simulink model "whatchman"  (R2013b)
settings: Solver=ode45  StartTime=0.0  StopTime=10  RelTol=1e-3
libraries: simulink_extras x4
settings Model: Creator=Maksimus  LastModifiedBy=Maksimus

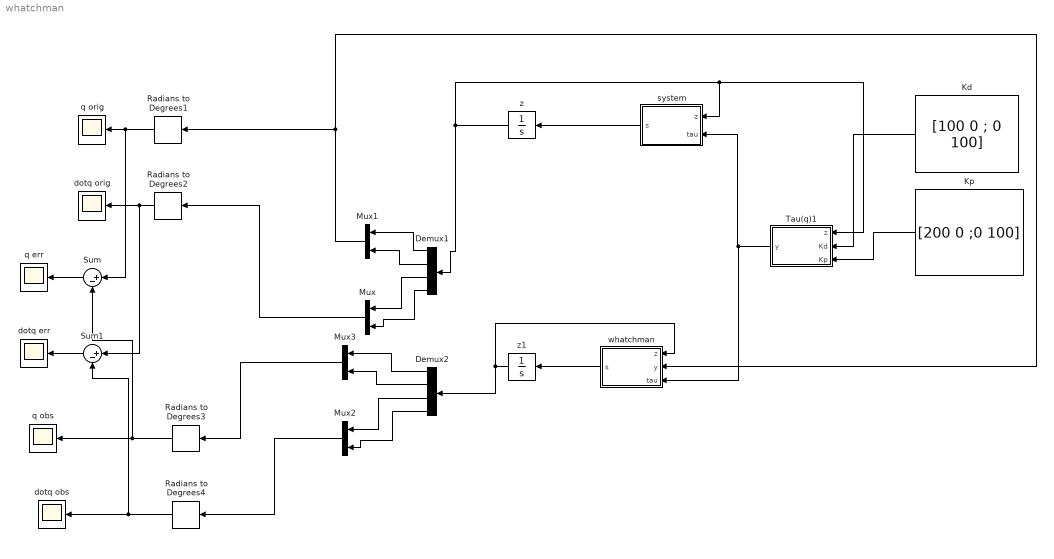
== system whatchman ==
  Demux1 : Demux
  Demux2 : Demux
  Kd : Constant  Value=[100 0 ; 0 100]
  "Kp " : Constant  Value=[200 0 ;0 100]
  Mux{,1..3} (4 alike) : Mux  Inputs=2
  Radians to Degrees{1..4} (4 alike) : simulink_extras/Transformations/Radians to Degrees
  Sum : Sum  Inputs=|+-
  Sum1 : Sum  Inputs=|+-
  Tau(q)1 : MATLAB Function  TreatAsAtomicUnit=on
  dotq err : Scope
      settings: YMin=0  YMax=30000  SaveName=ScopeData4
  dotq obs : Scope
      settings: YMin=0  YMax=30000
  dotq orig : Scope
      settings: YMin=0  YMax=30000  SaveName=ScopeData3
  q err : Scope
      settings: SaveName=ScopeData5
  q obs : Scope
  q orig : Scope
      settings: SaveName=ScopeData2
  system : MATLAB Function  TreatAsAtomicUnit=on
  whatchman : MATLAB Function  TreatAsAtomicUnit=on
  z : Integrator  InitialCondition=[0;0;0;0]  IgnoreLimit=on
  z1 : Integrator  InitialCondition=[-pi/2;0;0;0]  IgnoreLimit=on
  wires:
  Kd/1 -> Tau(q)1/2(Kd)
  z/1 -> Tau(q)1/1(z), system/1(z), Demux1/1
  Mux/1 -> Radians to Degrees2/1
  Demux1/1 -> Mux1/1
  Mux1/1 -> whatchman/2(y), Radians to Degrees1/1
  Radians to Degrees1/1 -> Sum/1, q orig/1
  Demux1/4 -> Mux/2
  Demux1/3 -> Mux/1
  system/1(s) -> z/1
  Tau(q)1/1(y) -> whatchman/3(tau), system/2(tau)
  "Kp "/1 -> Tau(q)1/3(Kp)
  Radians to Degrees2/1 -> Sum1/1, dotq orig/1
  Demux1/2 -> Mux1/2
  whatchman/1(s) -> z1/1
  z1/1 -> whatchman/1(z), Demux2/1
  Mux2/1 -> Radians to Degrees4/1
  Demux2/1 -> Mux3/1
  Mux3/1 -> Radians to Degrees3/1
  Radians to Degrees3/1 -> Sum/2, q obs/1
  Demux2/4 -> Mux2/2
  Demux2/3 -> Mux2/1
  Radians to Degrees4/1 -> Sum1/2, dotq obs/1
  Demux2/2 -> Mux3/2
  Sum1/1 -> dotq err/1
  Sum/1 -> q err/1

== matlab function whatchman/whatchman ==
  data: z input; y input; s output; tau input
function s = fcn(z,y,tau)
%задаем систему
m1 = 1; 
m2 = 1;
lc1 = 1;
lc2 = 2;
I1 = 0.12;
I2 = 0.12;
l1 = 1;
l2 = 1;
g=10;
m = [m1;m2];
lc = [lc1;lc2];
I = [I1;I2];
l = [l1;l2];
q = z(1:2);
dotq =z(3:4);

theta = [m(1)*lc(1)^2 + m(2)*l(1)^2 + I(1); m(2) * lc(2)^2 + I(2); m(2)*l(1)*lc(2); m(1)*lc(1) + m(2)*l(1); m(2)*lc(2)]; 

H = [theta(1) + theta(2) + 2 * theta(3)*cos(q(2)), theta(2) + theta(3) * cos(q(2));
    theta(2) + theta(3) * cos(q(2)), theta(2)]; 

C = [-theta(3) * sin(q(2)) * dotq(2), -theta(3) * sin(q(2)) * dotq(2) - theta(3) * sin(q(2)) * dotq(1);
    theta(3) * sin(q(2)) * dotq(1), 0];

G = [ theta(4) * g * cos(q(1)) + theta(5) * g * cos(q(1) + q(2)); theta(5) * g * cos(q(1) + q(2))]; %nonhorizontal robotarm
%конец задания системы


g1=15; %две константы, для того чтобы ошибка убывала
g2 = 210;

qcorrection =  g1* (y - q); %поправка для вектора углов
dotqcorrection =  g2*(y - q); %поправка для вектора скоростей
InvH = H^(-1);
InvHC = InvH * C;
InvHG = InvH * G;
tmpsys = - InvHC * dotq - InvHG + InvH*tau;
sys = [dotq + qcorrection ;tmpsys + dotqcorrection ]; 

s = sys;

== matlab function whatchman/system ==
  data: z input; s output; tau input
function s = fcn(z,tau)
%global linA linB linConst
%s = linA * z + linB * u + linConst;
m1 = 1;
m2 = 1;
lc1 = 1;
lc2 = 2;
I1 = 0.12;
I2 = 0.12;
l1 = 1;
l2 = 1;
g=10;

m = [m1;m2];
lc = [lc1;lc2];
I = [I1;I2];
l = [l1;l2];
dotq = z(3:4);
q = z(1:2);
theta = [m(1)*lc(1)^2 + m(2)*l(1)^2 + I(1); m(2) * lc(2)^2 + I(2); m(2)*l(1)*lc(2); m(1)*lc(1) + m(2)*l(1); m(2)*lc(2)]; 

H = [theta(1) + theta(2) + 2 * theta(3)*cos(q(2)), theta(2) + theta(3) * cos(q(2));
    theta(2) + theta(3) * cos(q(2)), theta(2)]; %is symmetrie, positive definite for all q

%H(q) - 2C(q, dotq) is a skew-syrnmetric matrix

C = [-theta(3) * sin(q(2)) * dotq(2), -theta(3) * sin(q(2)) * dotq(2) - theta(3) * sin(q(2)) * dotq(1);
    theta(3) * sin(q(2)) * dotq(1), 0];

G = [ theta(4) * g * cos(q(1)) + theta(5) * g * cos(q(1) + q(2)); theta(5) * g * cos(q(1) + q(2))]; %nonhorizontal robotarm


InvH = H^(-1);
InvHC = InvH * C;
InvHG = InvH * G;
tmpsys = - InvHC * dotq - InvHG + InvH*tau;
sys = [dotq;tmpsys];

s = sys;

== matlab function whatchman/Tau(q)1 ==
  data: z input; y output; Kd input; Kp input
function y = fcn(z, Kd, Kp)

qn = [30*pi/180; 90*pi/180];
qp  = z(1:2) - qn;
tau = -Kd * z(3:4) - Kp*qp;

y =tau;
